simulink model "gtm_design_baseline"  (Simulink 7.2)
settings: Solver=ode3  SolverMode=SingleTasking  StartTime=0.0  StopTime=Inf  FixedStep=Timestep  MaxStep=.1  RelTol=1e-5
StopFcn:
  | MWSout=grabmws(bdroot);
  | MWSout.lastrun=datestr(now);
model workspace: external: M-Code (data not in the file)
undefined symbols (not defined in the file or in its folder): alpha_trim, bias, CA, fc, invCB, Kb, Timestep, WindDir, WindSpd
libraries: simulink x3, aeroutilslib x2, aircraft_lib x1
CloseFcn:
  | rtwprivate ssgensfun ModelCloseRequest gtm_design
settings Model: Creator=cox  LastModifiedBy=E183308  ExtModeAutoUpdateStatusClock=off
settings DataIOCC: MaxDataPoints=50000  SaveFormat=Structure  SaveOutput=off  SignalLogging=off
settings OptimizationCC: BooleanDataType=off  InitFltsAndDblsToZero=on
settings DebuggingCC: SaveWithParameterizedLinksMsg=none  SignalResolutionControl=TryResolveAllWithWarning  SolverPrmCheckMsg=none  InheritedTsInSrcMsg=none  MultiTaskDSMMsg=warning  MultiTaskCondExecSysMsg=none  StrictBusMsg=None
settings HardwareCC: TargetHWDeviceType=32-bit Generic
settings RTWCC: IncludeERTFirstTime=on
settings GRTTargetCC: TargetFcnLib=ansi_tfl_tmw.mat

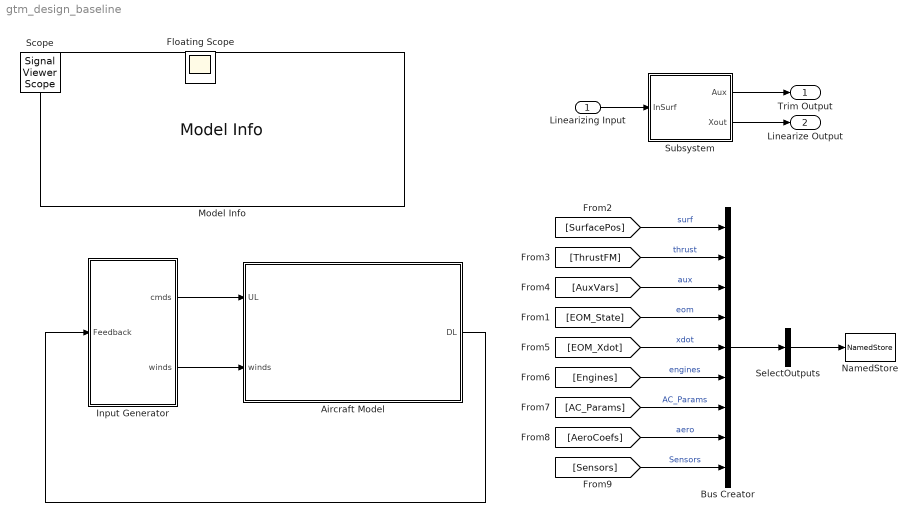
== system gtm_design_baseline ==
  Linearizing Input : Inport  OutDataType=sfix(16)  OutScaling=2^0
  Aircraft Model : Subsystem  BlockChoice=GTM_T2
      link override GTM_T2/Avionics: BlockChoice=Blank
      link override GTM_T2/Engines/GTM_T2/Bypass: Value=0
      link override GTM_T2/Sensors: BlockChoice=GTM_T2 gtm_design
      link override L1011_S2/Avionics: BlockChoice=Blank
      link override L1011_S2/Sensors: BlockChoice=Blank
      settings: AttributesFormatString=%<BlockChoice>  TemplateBlock=aircraft_lib/Aircraft Model  MemberBlocks=GTM_T2,L1011_S2
  Bus Creator : BusCreator  Inputs=9
  Input Generator : Subsystem
  Model Info : simulink/Model-Wide Utilities/Model Info  SystemSampleTime=-1  InitialBlockCM=none  BlockCM=none  Frame=on  DisplayStringWithTags=|  HorizontalTextAlignment=Center  LeftAlignmentValue=0.5  SourceBlockDiagram=gtm_design_baseline  TagMaxNumber=20
      | GTM Design-Simulation Model
      | Subversion Info: %<ModelVersion>
      | Last modified by %<LastModifiedBy> on %<LastModificationDate>
      | 
      | Copyright 2009
      | United States Government as represented by the 
      | Administrator of the National and Aeronautics and Space Administration.
      | 
      | No copyright is claimed in the United States under Title 17, U.S. Code.
      | All Other Rights Reserved.
  NamedStore : aeroutilslib/NamedStore  SystemSampleTime=-1  Npts=inf  VarName=sout  expand=off
  SelectOutputs : BusSelector  OutputSignals=aux.eas,aux.alpha,aux.beta,aux.gamma,surf.ELLOB,surf.ELLIB,surf.ELROB,surf.ELRIB  OutputAsBus=on
  Subsystem : Subsystem
  Trim Output : Outport  OutDataType=sfix(16)  OutScaling=2^0
  Linearize Output : Outport  Port=2  OutDataType=sfix(16)  OutScaling=2^0
  Floating Scope : Scope
      settings: Floating=on  YMin=0  YMax=7
  Scope : SignalViewerScope  IOType=viewer  RefreshTime=0.035000
  wires:
  SelectOutputs/1 -> NamedStore/1
  [SurfacePos] -> Bus Creator/1  "surf"
  Linearizing Input/1 -> Subsystem/1(InSurf)
  Subsystem/1(Aux) -> Trim Output/1
  [EOM_State] -> Bus Creator/4  "eom"
  [AuxVars] -> Bus Creator/3  "aux"
  [ThrustFM] -> Bus Creator/2  "thrust"
  Subsystem/2(Xout) -> Linearize Output/1
  [EOM_Xdot] -> Bus Creator/5  "xdot"
  [Engines] -> Bus Creator/6  "engines"
  [AC_Params] -> Bus Creator/7  "AC_Params"
  Bus Creator/1 -> SelectOutputs/1
  Input Generator/1(cmds) -> Aircraft Model/1(UL)
  Input Generator/2(winds) -> Aircraft Model/2(winds)
  Aircraft Model/1(DL) -> Input Generator/1(Feedback)
  [AeroCoefs] -> Bus Creator/8  "aero"
  [Sensors] -> Bus Creator/9  "Sensors"

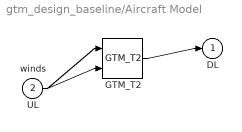
== system gtm_design_baseline/Aircraft Model ==
  UL : Inport  OutDataType=sfix(16)  OutScaling=2^0
  winds : Inport  Port=2  OutDataType=sfix(16)  OutScaling=2^0
  GTM_T2 : aircraft_lib/GTM_T2  Tag=From trunk/GTMsim/gtm_model.mdl revision 162  SystemSampleTime=-1
  DL : Outport  OutDataType=sfix(16)  OutScaling=2^0
  wires:
  UL/1 -> GTM_T2/1
  winds/1 -> GTM_T2/2
  GTM_T2/1 -> DL/1

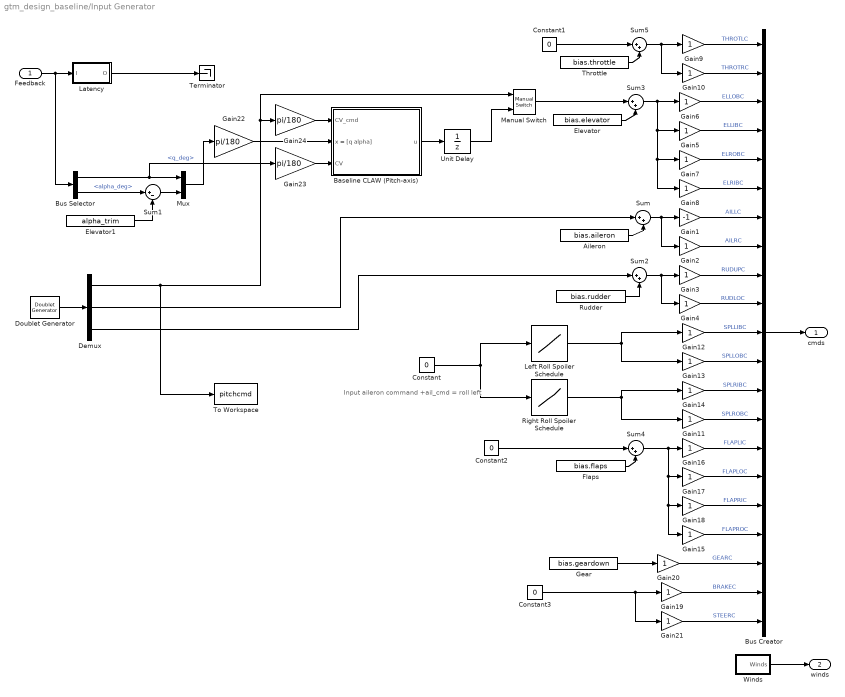
== system gtm_design_baseline/Input Generator ==
  note: Input aileron command
      | +ail_cmd = roll left
  Feedback : Inport  OutDataType=sfix(16)  OutScaling=2^0
  Aileron : Constant  Value=bias.aileron  OutDataType=sfix(16)  OutScaling=2^0
  Baseline CLAW (Pitch-axis) : Subsystem
  Bus Creator : BusCreator  Inputs=21
  Bus Selector : BusSelector  OutputSignals=MAG3.q_deg,AirData.alpha_deg
  Constant{,1..3} (4 alike) : Constant  Value=0  OutDataType=sfix(16)  OutScaling=2^0
  Demux : Demux  Outputs=3
  Doublet Generator : aeroutilslib/Doublet Generator  SystemSampleTime=-1  timeon=[2 0 0]  pulsewidth=[4 0 0]  amplitude=[0.500000 0.000000 0.000000]
  Elevator : Constant  Value=bias.elevator  OutDataType=sfix(16)  OutScaling=2^0
  Elevator1 : Constant  Value=alpha_trim  OutDataType=sfix(16)  OutScaling=2^0
  Flaps : Constant  Value=bias.flaps  OutDataType=sfix(16)  OutScaling=2^0
  Gain1 : Gain  Gain=-1  ParameterDataType=sfix(16)  ParameterScaling=2^0  OutDataType=sfix(16)  OutScaling=2^0  SaturateOnIntegerOverflow=on  OutDataTypeStr=Inherit: Same as input  ParamDataTypeStr=Inherit: Same as input
  Gain{2..21} (20 alike) : Gain  ParameterDataType=sfix(16)  ParameterScaling=2^0  OutDataType=sfix(16)  OutScaling=2^0  SaturateOnIntegerOverflow=on  OutDataTypeStr=Inherit: Same as input  ParamDataTypeStr=Inherit: Same as input
  Gain22 : Gain  Gain=pi/180  ParameterDataType=sfix(16)  ParameterScaling=2^0  OutDataType=sfix(16)  OutScaling=2^0  SaturateOnIntegerOverflow=on  OutDataTypeStr=Inherit: Same as input  ParamDataTypeStr=Inherit: Same as input
  Gain23 : Gain  Gain=pi/180  ParameterDataType=sfix(16)  ParameterScaling=2^0  OutDataType=sfix(16)  OutScaling=2^0  SaturateOnIntegerOverflow=on  OutDataTypeStr=Inherit: Same as input  ParamDataTypeStr=Inherit: Same as input
  Gain24 : Gain  Gain=pi/180  ParameterDataType=sfix(16)  ParameterScaling=2^0  OutDataType=sfix(16)  OutScaling=2^0  SaturateOnIntegerOverflow=on  OutDataTypeStr=Inherit: Same as input  ParamDataTypeStr=Inherit: Same as input
  Gear : Constant  Value=bias.geardown  OutDataType=sfix(16)  OutScaling=2^0
  Latency : Subsystem
  Left Roll Spoiler Schedule : Lookup  InputValues="[-20\t-11.76\t-2.36\t0\t2.36\t11.76\t20\t]"  Table=[0 0 0 0 0 9 45]  LookUpMeth=Interpolation-Use End Values  OutDataType=sfix(16)  OutScaling=2^0
  Manual Switch : simulink/Signal Routing/Manual Switch  SystemSampleTime=-1  sw=0  action=0  varsize=off
  Mux : Mux  Inputs=2
  Right Roll Spoiler Schedule : Lookup  InputValues="[-20\t-11.76\t-2.36\t0\t2.36\t11.76\t20\t]"  Table=[45 9 0 0 0 0 0]  LookUpMeth=Interpolation-Use End Values  OutDataType=sfix(16)  OutScaling=2^0
  Rudder : Constant  Value=bias.rudder  OutDataType=sfix(16)  OutScaling=2^0
  Sum{,2..5} (5 alike) : Sum  Inputs=|++  OutDataType=sfix(16)  OutScaling=2^0
  Sum1 : Sum  Inputs=|+-  OutDataType=sfix(16)  OutScaling=2^0
  Terminator : Terminator
  Throttle : Constant  Value=bias.throttle  OutDataType=sfix(16)  OutScaling=2^0
  To Workspace : ToWorkspace  VariableName=pitchcmd  SampleTime=-1  SaveFormat=Structure With Time
  Unit Delay : UnitDelay  SampleTime=Timestep
  Winds : Subsystem
  cmds : Outport  OutDataType=sfix(16)  OutScaling=2^0
  winds : Outport  Port=2  OutDataType=sfix(16)  OutScaling=2^0
  wires:
  Latency/1(O) -> Terminator/1
  Winds/1(Winds) -> winds/1
  Constant/1 -> Right Roll Spoiler Schedule/1, Left Roll Spoiler Schedule/1
  Right Roll Spoiler Schedule/1 -> Gain11/1, Gain14/1
  Left Roll Spoiler Schedule/1 -> Gain13/1, Gain12/1
  Gain12/1 -> Bus Creator/11  "SPLLIBC"
  Gain13/1 -> Bus Creator/12  "SPLLOBC"
  Gain14/1 -> Bus Creator/13  "SPLRIBC"
  Gain11/1 -> Bus Creator/14  "SPLROBC"
  Gain16/1 -> Bus Creator/15  "FLAPLIC"
  Gain17/1 -> Bus Creator/16  "FLAPLOC"
  Gain18/1 -> Bus Creator/17  "FLAPRIC"
  Gain15/1 -> Bus Creator/18  "FLAPROC"
  Gain9/1 -> Bus Creator/1  "THROTLC"
  Gain10/1 -> Bus Creator/2  "THROTRC"
  Gain5/1 -> Bus Creator/4  "ELLIBC"
  Gain6/1 -> Bus Creator/3  "ELLOBC"
  Gain7/1 -> Bus Creator/5  "ELROBC"
  Gain8/1 -> Bus Creator/6  "ELRIBC"
  Gain1/1 -> Bus Creator/7  "AILLC"
  Gain2/1 -> Bus Creator/8  "AILRC"
  Gain3/1 -> Bus Creator/9  "RUDUPC"
  Gain4/1 -> Bus Creator/10  "RUDLOC"
  Throttle/1 -> Sum5/2
  Constant1/1 -> Sum5/1
  Sum5/1 -> Gain10/1, Gain9/1
  Sum3/1 -> Gain6/1, Gain5/1, Gain7/1, Gain8/1
  Aileron/1 -> Sum/2
  Elevator/1 -> Sum3/2
  Sum/1 -> Gain1/1, Gain2/1
  Sum2/1 -> Gain3/1, Gain4/1
  Rudder/1 -> Sum2/2
  Flaps/1 -> Sum4/2
  Constant2/1 -> Sum4/1
  Sum4/1 -> Gain16/1, Gain17/1, Gain18/1, Gain15/1
  Doublet Generator/1 -> Demux/1
  Demux/2 -> Sum/1
  Demux/3 -> Sum2/1
  Gain19/1 -> Bus Creator/20  "BRAKEC"
  Gear/1 -> Gain20/1
  Constant3/1 -> Gain19/1, Gain21/1
  Bus Creator/1 -> cmds/1
  Feedback/1 -> Latency/1(I), Bus Selector/1
  Gain20/1 -> Bus Creator/19  "GEARC"
  Gain21/1 -> Bus Creator/21  "STEERC"
  Demux/1 -> Manual Switch/1, Gain24/1, To Workspace/1
  Manual Switch/1 -> Sum3/1
  Baseline CLAW (Pitch-axis)/1(u) -> Unit Delay/1
  Bus Selector/1 -> Mux/1, Gain23/1  "<q_deg>"
  Mux/1 -> Gain22/1
  Gain22/1 -> Baseline CLAW (Pitch-axis)/2(x = [q alpha])
  Gain23/1 -> Baseline CLAW (Pitch-axis)/3(CV)
  Gain24/1 -> Baseline CLAW (Pitch-axis)/1(CV_cmd)
  Bus Selector/2 -> Sum1/1  "<alpha_deg>"
  Sum1/1 -> Mux/2
  Elevator1/1 -> Sum1/2
  Unit Delay/1 -> Manual Switch/2

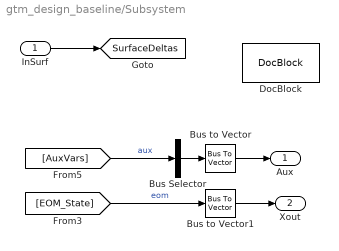
== system gtm_design_baseline/Subsystem ==
  InSurf : Inport  OutDataType=sfix(16)  OutScaling=2^0
  Bus Selector : BusSelector  OutputSignals=eas,tas,alpha,beta,gamma,gndtrack  OutputAsBus=on
  Bus to Vector : BusToVector
  Bus to Vector1 : BusToVector
  DocBlock : simulink/Model-Wide Utilities/DocBlock  SystemSampleTime=-1  DocumentType=Text
      content=|
      | Inputs and Outputs selected here have a specific ordering.
      |
      |
      |
      | Do not change this without also changing output channel ordering in associated linmodel.m and
      | trimgtm.m functions
  Aux : Outport  OutDataType=sfix(16)  OutScaling=2^0
  Xout : Outport  Port=2  OutDataType=sfix(16)  OutScaling=2^0
  tag scope: SurfaceDeltas=global
  wires:
  [AuxVars] -> Bus Selector/1  "aux"
  [EOM_State] -> Bus to Vector1/1  "eom"
  Bus Selector/1 -> Bus to Vector/1
  InSurf/1 -> [SurfaceDeltas]
  Bus to Vector/1 -> Aux/1
  Bus to Vector1/1 -> Xout/1

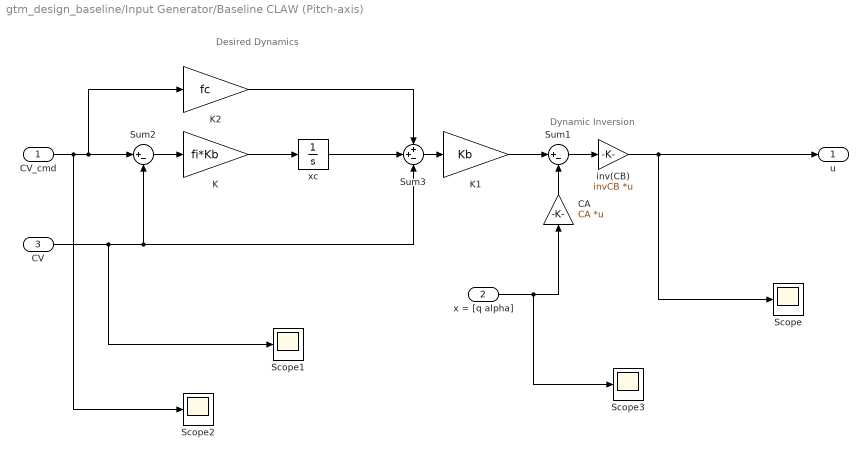
== system gtm_design_baseline/Input Generator/Baseline CLAW (Pitch-axis) ==
  note: Desired
      | Dynamics
  note: Dynamic
      | Inversion
  CV_cmd : Inport  OutDataType=sfix(16)  OutScaling=2^0
  x = [q alpha] : Inport  Port=2  OutDataType=sfix(16)  OutScaling=2^0
  CV : Inport  Port=3  OutDataType=sfix(16)  OutScaling=2^0
  CA : Gain  Orientation=up  Gain=CA  Multiplication=Matrix(K*u)  ParameterDataType=sfix(16)  ParameterScaling=2^0  OutDataType=sfix(16)  OutScaling=2^0
  K : Gain  Gain=fi*Kb  ParameterDataType=sfix(16)  ParameterScaling=2^0  OutDataType=sfix(16)  OutScaling=2^0
  K1 : Gain  Gain=Kb  ParameterDataType=sfix(16)  ParameterScaling=2^0  OutDataType=sfix(16)  OutScaling=2^0
  K2 : Gain  Gain=fc  ParameterDataType=sfix(16)  ParameterScaling=2^0  OutDataType=sfix(16)  OutScaling=2^0
  Scope{,1..3} (4 alike) : Scope
      Scope settings: YMin=-1e-009  YMax=1e-010
      Scope1 settings: SaveName=ScopeData2
      Scope2 settings: SaveName=ScopeData3
      Scope3 settings: SaveName=ScopeData4
  Sum1 : Sum  Inputs=|+-  OutDataType=sfix(16)  OutScaling=2^0
  Sum2 : Sum  Inputs=|+-  OutDataType=sfix(16)  OutScaling=2^0
  Sum3 : Sum  Inputs=++-  OutDataType=sfix(16)  OutScaling=2^0
  inv(CB) : Gain  Gain=invCB  Multiplication=Matrix(K*u)  ParameterDataType=sfix(16)  ParameterScaling=2^0  OutDataType=sfix(16)  OutScaling=2^0
  xc : Integrator
  u : Outport  OutDataType=sfix(16)  OutScaling=2^0
  wires:
  Sum1/1 -> inv(CB)/1
  CA/1 -> Sum1/2
  CV_cmd/1 -> Sum2/1, K2/1, Scope2/1
  inv(CB)/1 -> Scope/1, u/1
  x = [q alpha]/1 -> CA/1, Scope3/1
  K/1 -> xc/1
  Sum2/1 -> K/1
  xc/1 -> Sum3/2
  CV/1 -> Sum2/2, Sum3/3, Scope1/1
  Sum3/1 -> K1/1
  K2/1 -> Sum3/1
  K1/1 -> Sum1/1

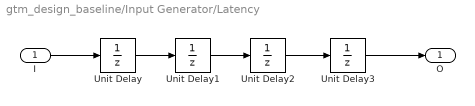
== system gtm_design_baseline/Input Generator/Latency ==
  I : Inport  OutDataType=sfix(16)  OutScaling=2^0
  Unit Delay{,1..3} (4 alike) : UnitDelay  SampleTime=Timestep
  O : Outport  OutDataType=sfix(16)  OutScaling=2^0
  wires:
  Unit Delay3/1 -> O/1
  Unit Delay2/1 -> Unit Delay3/1
  Unit Delay1/1 -> Unit Delay2/1
  Unit Delay/1 -> Unit Delay1/1
  I/1 -> Unit Delay/1

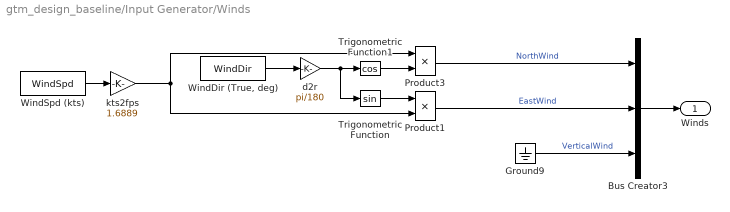
== system gtm_design_baseline/Input Generator/Winds ==
  Bus Creator3 : BusCreator  Inputs=3
  Ground9 : Ground
  Product1 : Product  Inputs=**  OutDataType=sfix(16)  OutScaling=2^0  SaturateOnIntegerOverflow=on  InputSameDT=on  OutDataTypeStr=Inherit: Same as first input
  Product3 : Product  Inputs=**  OutDataType=sfix(16)  OutScaling=2^0  SaturateOnIntegerOverflow=on  InputSameDT=on  OutDataTypeStr=Inherit: Same as first input
  Trigonometric Function : Trigonometry
  Trigonometric Function1 : Trigonometry  Operator=cos
  "WindDir (True, deg)" : Constant  Value=WindDir  OutDataType=sfix(16)  OutScaling=2^0
  WindSpd (kts) : Constant  Value=WindSpd  OutDataType=sfix(16)  OutScaling=2^0
  d2r : Gain  Gain=pi/180  ParameterDataType=sfix(16)  ParameterScaling=2^0  OutDataType=sfix(16)  OutScaling=2^0  SaturateOnIntegerOverflow=on  OutDataTypeStr=Inherit: Same as input  ParamDataTypeStr=Inherit: Same as input
  kts2fps : Gain  Gain=1.6889  ParameterDataType=sfix(16)  ParameterScaling=2^0  OutDataType=sfix(16)  OutScaling=2^0  SaturateOnIntegerOverflow=on  OutDataTypeStr=Inherit: Same as input  ParamDataTypeStr=Inherit: Same as input
  Winds : Outport  OutDataType=sfix(16)  OutScaling=2^0
  wires:
  kts2fps/1 -> Product1/2, Product3/1
  WindSpd (kts)/1 -> kts2fps/1
  "WindDir (True, deg)"/1 -> d2r/1
  d2r/1 -> Trigonometric Function1/1, Trigonometric Function/1
  Trigonometric Function1/1 -> Product3/2
  Trigonometric Function/1 -> Product1/1
  Bus Creator3/1 -> Winds/1
  Ground9/1 -> Bus Creator3/3  "VerticalWind"
  Product1/1 -> Bus Creator3/2  "EastWind"
  Product3/1 -> Bus Creator3/1  "NorthWind"
